simulink model "LuGre_Model"  (R2023b)
settings: Solver=VariableStepAuto  StartTime=0.0  StopTime=10.0  RelTol=1e-3
settings Model: Creator=hp  LastModifiedBy=hp

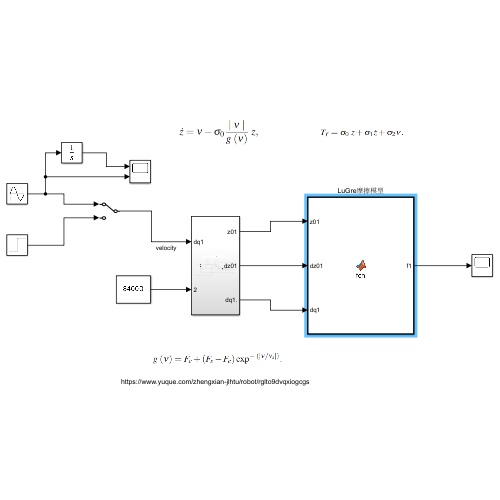
[thumbnail: Simulink's stored preview of the top-level diagram]
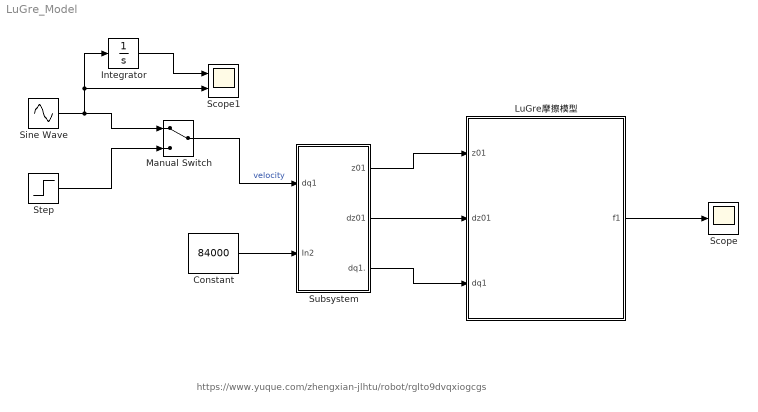
== system LuGre_Model ==
  note: https://www.yuque.com/zhengxian-jlhtu/robot/rglto9dvqxiogcgs
  Constant : Constant  Value=84000
  Integrator : Integrator
  LuGre摩擦模型 : MATLAB Function  TreatAsAtomicUnit=on
  Manual Switch : ManualSwitch
  Scope : Scope
  Scope1 : Scope  NumInputPorts=2
  Sine Wave : Sin  SampleTime=0
  Step : Step  SampleTime=0
  Subsystem : Subsystem
  wires:
  Constant/1 -> Subsystem/2(In2)
  Subsystem/1(z01) -> LuGre摩擦模型/1(z01)
  Subsystem/2(dz01) -> LuGre摩擦模型/2(dz01)
  Subsystem/3(dq1.) -> LuGre摩擦模型/3(dq1)
  LuGre摩擦模型/1(f1) -> Scope/1
  Step/1 -> Manual Switch/2
  Sine Wave/1 -> Manual Switch/1, Integrator/1, Scope1/2
  Manual Switch/1 -> Subsystem/1(dq1)  "velocity"
  Integrator/1 -> Scope1/1

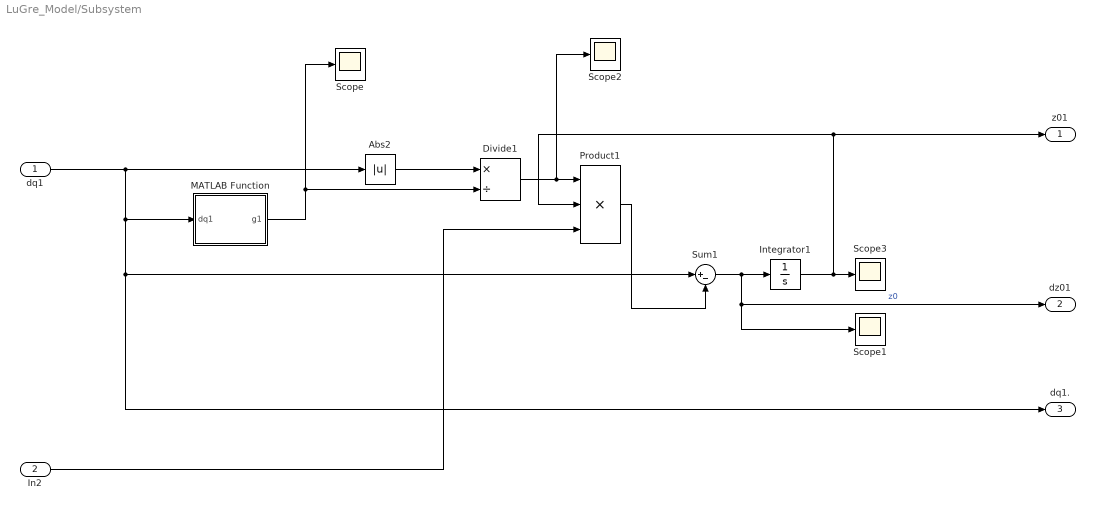
== system LuGre_Model/Subsystem ==
  dq1 : Inport
  In2 : Inport  Port=2
  Abs2 : Abs  SaturateOnIntegerOverflow=off
  Divide1 : Product  Inputs=*/
  Integrator1 : Integrator
  MATLAB Function : MATLAB Function  TreatAsAtomicUnit=on
  Product1 : Product  Inputs=3
  Scope{,1..3} (4 alike) : Scope
  Sum1 : Sum  Inputs=|+-
  z01 : Outport
  dz01 : Outport  Port=2
  dq1. : Outport  Port=3
  wires:
  Abs2/1 -> Divide1/1
  In2/1 -> Product1/3
  Sum1/1 -> dz01/1, Scope1/1, Integrator1/1  "z0"
  Integrator1/1 -> Scope3/1, z01/1, Product1/2
  MATLAB Function/1(g1) -> Scope/1, Divide1/2
  dq1/1 -> MATLAB Function/1(dq1), dq1./1, Sum1/1, Abs2/1
  Product1/1 -> Sum1/2
  Divide1/1 -> Scope2/1, Product1/1

== matlab function LuGre_Model/LuGre摩擦模型 ==
  data: z01 input; dz01 input; dq1 input; f1 output
function f1  = fcn(z01,dz01,dq1)
xite0 = 84000;
xite1 = 260;
xite2 = 28;
Fc = 3.82;
Fs = 8.16;
dqs = 0.0125;
lamda = 0.1;

f1 = lamda * (xite0 * z01 + xite1 * dz01 + xite2 * dq1);

== matlab function LuGre_Model/Subsystem/MATLAB Function ==
  data: dq1 input; g1 output
function g1 = fcn(dq1)
xite1 = 260;
xite2 = 28;
Fc = 3.82;
Fs = 8.16;
dqs = 0.0125;

g1 = Fc + (Fs-Fc)*exp(-(dq1/dqs)^2);
